simulink model "sla_QPSK"  (R2015b)
settings: Solver=FixedStepDiscrete  SolverMode=SingleTasking  StartTime=0.0  StopTime=0.1  RelTol=1e-3
PreLoadFcn:
  | EbNo=100
  | maxNumErrs=1
  | maxNumBits=1
undefined symbols (not defined in the file or in its folder): M, rcosine
libraries: dspobslib x2, commdigbbndpm3 x2, commcnvcod2 x2, commchan3 x1, commrandsrc2 x1, commsink2 x1
settings Model: Creator=at-mt  LastModifiedBy=amatsumo
settings DataIOCC: SaveFormat=Array  SignalLoggingSaveFormat=ModelDataLogs  SaveOutput=off  SignalLogging=off  SaveTime=off
settings OptimizationCC: BlockReduction=off  ConditionallyExecuteInputs=off  DefaultParameterBehavior=Inlined  ExpressionDepthLimit=2147483647
settings DebuggingCC: AlgebraicLoopMsg=error  UnderspecifiedInitializationDetection=Classic  MergeDetectMultiDrivingBlocksExec=none  SolverPrmCheckMsg=warning  SingleTaskRateTransMsg=error  ParameterPrecisionLossMsg=none  FcnCallInpInsideContextMsg=UseLocalSettings  StateNameClashWarn=warning
settings HardwareCC: ProdBitPerPointer=32  ProdLargestAtomicFloat=None  ProdIntDivRoundTo=Undefined  ProdEndianess=Unspecified  ProdWordSize=32  ProdHWDeviceType=ASIC/FPGA->ASIC/FPGA  ProdEqTarget=off
settings GRTTargetCC: GeneratePreprocessorConditionals=Disable all  CombineOutputUpdateFcns=off  GRTInterface=on
settings ConfigComp: CovModelRefEnable=Off  CovSFcnEnable=off

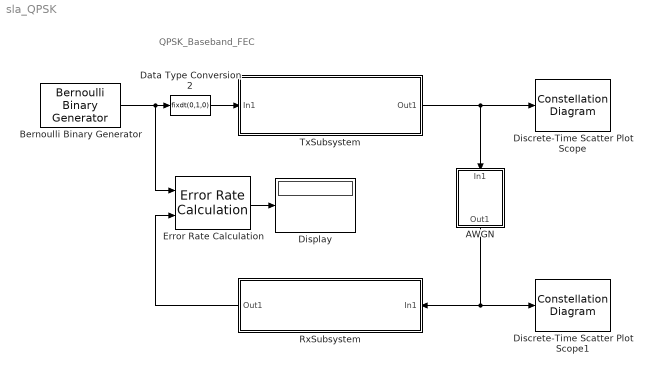
== system sla_QPSK ==
  note: QPSK_Baseband_FEC
  AWGN : Subsystem
  Bernoulli Binary Generator : commrandsrc2/Bernoulli Binary Generator  P=0.5  seed=randseed  Ts=1e-6/log2(4)  frameBased=off  sampPerFrame=1  orient=off  outDataType=boolean
  Data Type Conversion2 : DataTypeConversion  OutDataTypeStr=fixdt(0,1,0)
  Discrete-Time Scatter Plot Scope : ConstellationDiagram  Tag=ScatterPlot
  Discrete-Time Scatter Plot Scope1 : ConstellationDiagram  Tag=ScatterPlot
  Display : Display
  Error Rate Calculation : commsink2/Error Rate Calculation  N=4+4+34+6  st_delay=0  cp_mode=Entire frame  subframe=[]  PMode=Port  WsName=BER  RsMode2=off  stop=off  numErr=maxNumErrs  maxBits=maxNumBits
  RxSubsystem : Subsystem
  TxSubsystem : Subsystem
  wires:
  Bernoulli Binary Generator/1 -> Data Type Conversion2/1, Error Rate Calculation/1
  Error Rate Calculation/1 -> Display/1
  RxSubsystem/1(Out1) -> Error Rate Calculation/2
  Data Type Conversion2/1 -> TxSubsystem/1(In1)
  TxSubsystem/1(Out1) -> Discrete-Time Scatter Plot Scope/1, AWGN/1(In1)
  AWGN/1(Out1) -> Discrete-Time Scatter Plot Scope1/1, RxSubsystem/1(In1)

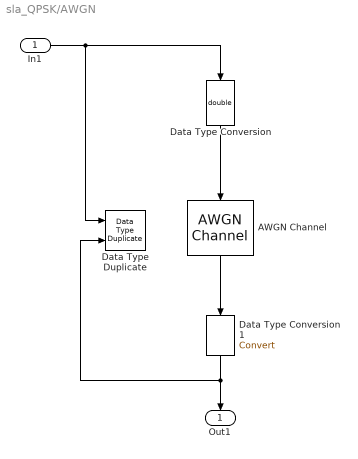
== system sla_QPSK/AWGN ==
  In1 : Inport
  AWGN Channel : commchan3/AWGN Channel  InputProcessing=Inherited (this choice will be removed - see release notes)  seed=randseed  noiseMode="Signal to noise ratio  (Eb/No)"  EbNodB=EbNo+10*log10(1/2)  EsNodB=10  SNRdB=EbNo+10*log10(log2(M))-10*log10((1e-6)/(1e-6))  bitsPerSym=log2(4)  Ps=0.125  Tsym=(1e-6)/2  variance=1
  Data Type Duplicate : DataTypeDuplicate
  Data Type Conversion : DataTypeConversion  OutDataTypeStr=double
  Data Type Conversion1 : DataTypeConversion
  Out1 : Outport
  wires:
  AWGN Channel/1 -> Data Type Conversion1/1
  Data Type Conversion/1 -> AWGN Channel/1
  In1/1 -> Data Type Conversion/1, Data Type Duplicate/1
  Data Type Conversion1/1 -> Out1/1, Data Type Duplicate/2

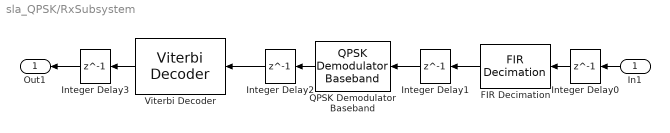
== system sla_QPSK/RxSubsystem ==
  In1 : Inport
  FIR Decimation : dspobslib/FIR Decimation  FilterSource=Dialog parameters  h=rcosine(1,8,'sqrt',0.5,4)  D=8  filtStruct=Direct form  FilterObject=Hm_firdecim  InputProcessing=Inherited (this choice will be removed - see release notes)  framing=Allow multirate processing  inputOffset=0  outputBufInitCond=0  roundingMode=Floor  overflowMode=off  firstCoeffMode=Specify word length  firstCoeffWordLength=16  firstCoeffFracLength=16  firstCoeffDataTypeStr=fixdt(1,16)  firstCoeffMin=[]  firstCoeffMax=[]  firstCoeffLastDataTypeStr=fixdt(1,16)  prodOutputMode=Binary point scaling  prodOutputWordLength=16  prodOutputFracLength=15  prodOutputDataTypeStr=fixdt(1,16,15)  prodOutputLastDataTypeStr=fixdt(1,16,15)  accumMode=Binary point scaling  accumWordLength=24  accumFracLength=20  accumDataTypeStr=fixdt(1,24,20)  accumLastDataTypeStr=fixdt(1,24,20)  outputMin=[]  outputMax=[]
  Integer Delay{0..3} (4 alike) : Delay  DelayLength=1
  QPSK Demodulator Baseband : commdigbbndpm3/QPSK Demodulator Baseband  Ph=pi/4  Dec=Gray  OutType=Bit  DecType=Hard decision  VarSource=Dialog  Variance=1  outDtype1=Smallest unsigned integer  outDtype2=double  derotateFactorDTMode=Specify word length  derotateFactorWordLen=16
  Viterbi Decoder : commcnvcod2/Viterbi Decoder  trellis=poly2trellis(7, [171 133])  isPunctured=off  punctureVector=[1; 1; 0; 1; 0; 1]  erasures=off  dectype=Hard decision  runSigValErrCheck=off  nsdecb=4  smWordLength=5  tbdepth=34  opmode=Continuous  reset=off  outDataType=boolean  delayedResetAction=off
  Out1 : Outport
  wires:
  QPSK Demodulator Baseband/1 -> Integer Delay2/1
  FIR Decimation/1 -> Integer Delay1/1
  In1/1 -> Integer Delay0/1
  Viterbi Decoder/1 -> Integer Delay3/1
  Integer Delay0/1 -> FIR Decimation/1
  Integer Delay1/1 -> QPSK Demodulator Baseband/1
  Integer Delay2/1 -> Viterbi Decoder/1
  Integer Delay3/1 -> Out1/1

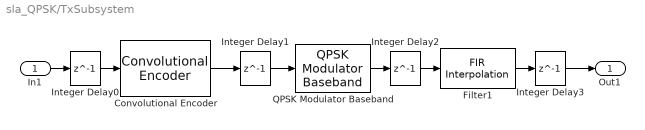
== system sla_QPSK/TxSubsystem ==
  In1 : Inport
  Convolutional Encoder : commcnvcod2/Convolutional Encoder  trellis=poly2trellis(7, [171 133])  opMode=Continuous  DelayedResetAction=off  hasIniStPort=off  hasFinStPort=off  usePuncVector=off  punctureVector=[1; 1; 0; 1; 0; 1]  reset=Unused parameter value
  Filter1 : dspobslib/FIR Interpolation  Tag=BlockMethodSubSystem  FilterSource=Dialog parameters  h=rcosine(1,8,'sqrt',0.5,4)  L=8  FilterObject=Hm_firinterp  InputProcessing=Inherited (this choice will be removed - see release notes)  framing=Allow multirate processing  outputBufInitCond=0  roundingMode=Floor  overflowMode=off  firstCoeffMode=Specify word length  firstCoeffWordLength=16  firstCoeffFracLength=16  firstCoeffDataTypeStr=fixdt(1,16)  firstCoeffMin=[]  firstCoeffMax=[]  firstCoeffLastDataTypeStr=fixdt(1,16)  prodOutputMode=Binary point scaling  prodOutputWordLength=16  prodOutputFracLength=15  prodOutputDataTypeStr=fixdt(1,16,15)  prodOutputLastDataTypeStr=fixdt(1,16,15)  accumMode=Binary point scaling  accumWordLength=24  accumFracLength=21  accumDataTypeStr=fixdt(1,24,21)  accumLastDataTypeStr=fixdt(1,24,21)  outputMin=[]  outputMax=[]
  Integer Delay{0..3} (4 alike) : Delay  DelayLength=1
  QPSK Modulator Baseband : commdigbbndpm3/QPSK Modulator Baseband  InType=Bit  Enc=Gray  Ph=pi/4  outDtype=Fixed-point  outWordLen=16  outUDDataType=sfix(16)  outFracLenMode=Best precision  outFracLen=15
  Out1 : Outport
  wires:
  In1/1 -> Integer Delay0/1
  QPSK Modulator Baseband/1 -> Integer Delay2/1
  Convolutional Encoder/1 -> Integer Delay1/1
  Filter1/1 -> Integer Delay3/1
  Integer Delay0/1 -> Convolutional Encoder/1
  Integer Delay1/1 -> QPSK Modulator Baseband/1
  Integer Delay2/1 -> Filter1/1
  Integer Delay3/1 -> Out1/1
